simulink model "Ex10_5_ResponseWithADeadZone"  (R2023a)
settings: Solver=VariableStepAuto  StartTime=0.0  StopTime=10.0  RelTol=1e-3
settings Model: Creator=Norb  LastModifiedBy=Norb

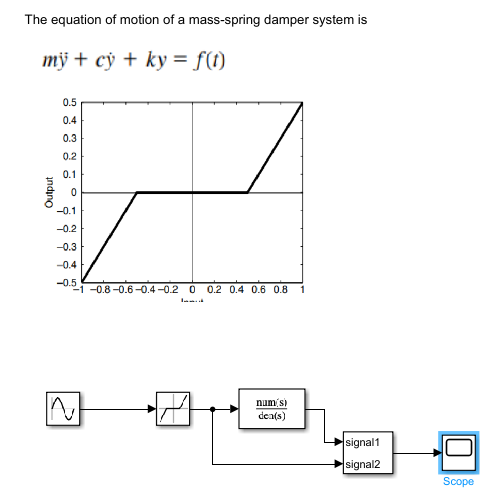
[thumbnail: Simulink's stored preview of the top-level diagram]
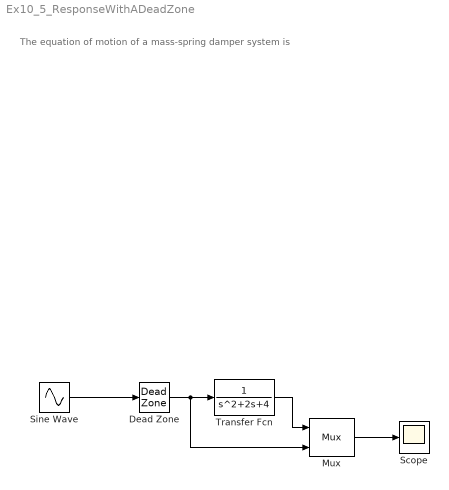
== system Ex10_5_ResponseWithADeadZone ==
  note: The equation of motion of a mass-spring damper system is
  Dead Zone : DeadZone
  Mux : Mux  Inputs=2
      settings: DisplayOption=signals
  Scope : Scope
  Sine Wave : Sin  Frequency=1.4  SampleTime=0
  Transfer Fcn : TransferFcn  Denominator=[1,2,4]
  wires:
  Sine Wave/1 -> Dead Zone/1
  Dead Zone/1 -> Mux/2, Transfer Fcn/1
  Transfer Fcn/1 -> Mux/1
  Mux/1 -> Scope/1
